simulink model "Simulink_EbolaControlMIMO"  (R2021b)
settings: Solver=VariableStepAuto  StartTime=0.0  StopTime=100  FixedStep=0.0447626744587381  RelTol=1e-3
model workspace (MAT data in the model file):
  Beta = 1.905e-07
  C = 8.015
  Delta = 0.001
  P = 378
  U = 500
  Uu = 250
  V0 = 1.05
  u = 500
undefined symbols (not defined in the file or in its folder): sigbuilder_block
settings Model: Creator=Camilo  LastModifiedBy=Camilo
settings DataIOCC: SaveFormat=Array  OutputTimes=tout

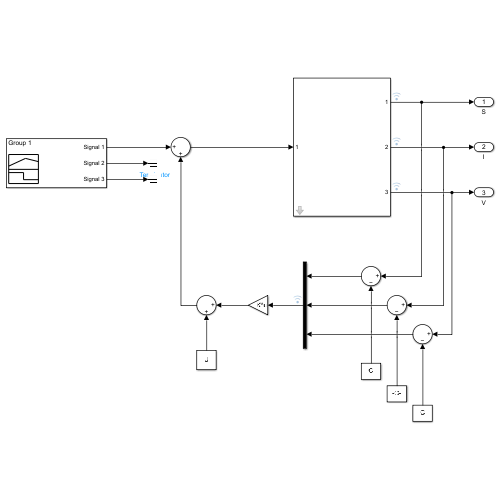
[thumbnail: Simulink's stored preview of the top-level diagram]
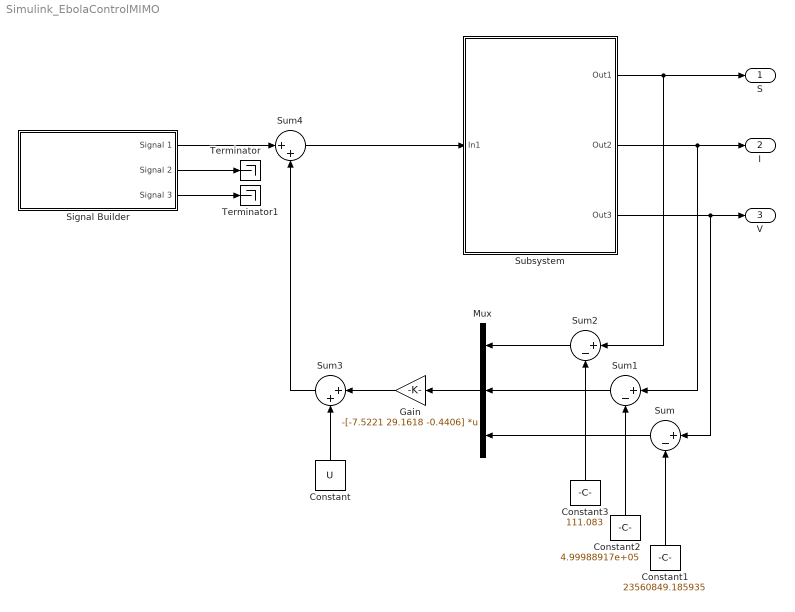
== system Simulink_EbolaControlMIMO ==
  Constant : Constant  Value=U  mask{U=0}
  Constant1 : Constant  Value=23560849.185935
  Constant2 : Constant  Value=4.99988917e+05
  Constant3 : Constant  Value=111.083
  Gain : Gain  Gain=-[-7.5221 29.1618 -0.4406]  Multiplication=Matrix(K*u)
  Mux : Mux  Inputs=3
  Signal Builder : Subsystem  Tag=STV Subsys  LoadFcn=sigbuilder_block('load');  StartFcn=sigbuilder_block('start');  StopFcn=sigbuilder_block('stop');  ClipboardFcn=sigbuilder_block('clipboard');  mask(Sigbuilder block){tuvar=[0:10]}
      mask help: Simulink:masks:SigbuilderBlock_MD
      mask init:
      | if ~strcmp(get_param(bdroot(gcbh),'SimulationStatus'),'stopped') tuvar = sigbuilder_block('maskInit'); end
      settings: CopyFcn=sigbuilder_block('copy');  DeleteFcn=sigbuilder_block('delete');  ModelCloseFcn=sigbuilder_block('modelClose');  PreSaveFcn=sigbuilder_block('preSave');  PauseFcn=sigbuilder_block('pause');  ContinueFcn=sigbuilder_block('continue');  NameChangeFcn=sigbuilder_block('namechange');  OpenFcn=sigbuilder_block('open',[437.6 126.75 619.15 472.45 ]);  CloseFcn=sigbuilder_block('close');
      mask Display: plot(0, 0, 100, 100,[2, 2, 32, 32, 2], [68, 8, 8, 68, 68],[32, 2], [38, 38], [32, 19, 2],[53, 60, 44], [32, 17, 17, 2],[16, 16, 31, 31]);txt = getActiveGroup(gcbh);text(2, 100, txt,'verticalAlignment', 'top');
  Subsystem : Subsystem  mask{V0=23560849.185935, Delta=Delta, P=P, C=C, Beta=Beta}
  Sum : Sum  Inputs=|+-
  Sum1 : Sum  Inputs=|+-
  Sum2 : Sum  Inputs=|+-
  Sum3 : Sum  Inputs=|++
  Sum4 : Sum  Inputs=|++
  Terminator : Terminator
  Terminator1 : Terminator
  S : Outport
  I : Outport  Port=2
  V : Outport  Port=3
  wires:
  Subsystem/2(Out2) -> I/1, Sum1/1
  Subsystem/3(Out3) -> V/1, Sum/1
  Subsystem/1(Out1) -> Sum2/1, S/1
  Constant1/1 -> Sum/2
  Constant2/1 -> Sum1/2
  Constant3/1 -> Sum2/2
  Sum/1 -> Mux/3
  Sum2/1 -> Mux/1
  Sum1/1 -> Mux/2
  Mux/1 -> Gain/1
  Gain/1 -> Sum3/1
  Constant/1 -> Sum3/2
  Sum3/1 -> Sum4/2
  Sum4/1 -> Subsystem/1(In1)
  Signal Builder/1(Signal 1) -> Sum4/1
  Signal Builder/3(Signal 3) -> Terminator1/1
  Signal Builder/2(Signal 2) -> Terminator/1

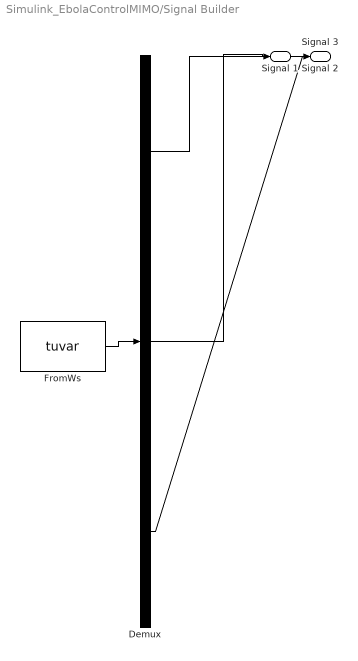
== system Simulink_EbolaControlMIMO/Signal Builder ==
  Demux : Demux  Tag=STV Demux  Outputs=3
      settings: DisplayOption=none
  FromWs : FromWorkspace  Tag=STV FromWs  VariableName=tuvar
      SigBuilderData=|
      | common.afterFinalStr = 'Extrapolate'
      | common.sampleTime = 0
      | dataSet.timeRange = [0 10]
      | dataSet.name = 'Group 1'
      | sbobj.Groups.Name = 'Group 1'
      | sbobj.Groups.Signals(1).Name = 'Signal 1'
      | sbobj.Groups.Signals(1).XData = [0 3 6 6 10]
      | sbobj.Groups.Signals(1).YData = [0.01 0 500 -0.005 0]
      | sbobj.Groups.Signals(2).Name = 'Signal 2'
      | sbobj.Groups.Signals(2).XData = [0 4 4 10]
      | sbobj.Groups.Signals(2).YData = [0 0 500 500]
      | sbobj.Groups.Signals(3).Name = 'Signal 3'
      | sbobj.Groups.Signals(3).XData = [0 4 4 6 6 10]
      | sbobj.Groups.Signals(3).YData = [0 0 500 500 0 0]
  Signal 1 : Outport  Tag=STV Outport
  Signal 2 : Outport  Tag=STV Outport  Port=2
  Signal 3 : Outport  Tag=STV Outport  Port=3
  wires:
  Demux/1 -> Signal 1/1
  FromWs/1 -> Demux/1
  Demux/2 -> Signal 2/1
  Demux/3 -> Signal 3/1

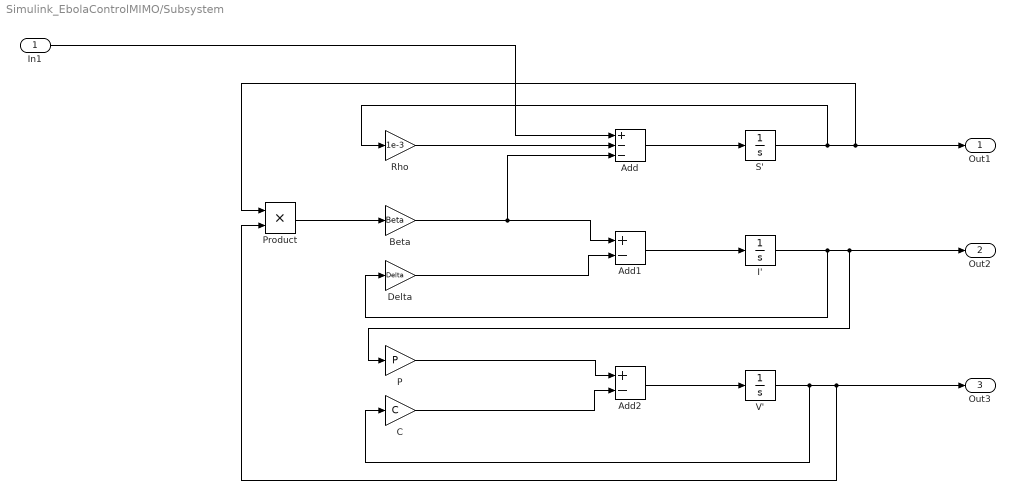
== system Simulink_EbolaControlMIMO/Subsystem ==
  In1 : Inport
  Add : Sum  Inputs=+--
  Add1 : Sum  Inputs=+-
  Add2 : Sum  Inputs=+-
  Beta : Gain  Gain=Beta
  C : Gain  Gain=C
  Delta : Gain  Gain=Delta
  I' : Integrator  InitialCondition=4.99988917e5  LimitOutput=on  LowerSaturationLimit=0
  P : Gain  Gain=P
  Product : Product
  Rho : Gain  Gain=1e-3
  S' : Integrator  InitialCondition=111.083  LimitOutput=on  LowerSaturationLimit=0
  V' : Integrator  InitialCondition=V0  LimitOutput=on  LowerSaturationLimit=0
  Out1 : Outport
  Out2 : Outport  Port=2
  Out3 : Outport  Port=3
  wires:
  Add/1 -> S'/1
  C/1 -> Add2/2
  Beta/1 -> Add1/1, Add/3
  I'/1 -> Out2/1, P/1, Delta/1
  P/1 -> Add2/1
  S'/1 -> Out1/1, Product/1, Rho/1
  Rho/1 -> Add/2
  V'/1 -> Out3/1, Product/2, C/1
  Add2/1 -> V'/1
  Product/1 -> Beta/1
  Add1/1 -> I'/1
  Delta/1 -> Add1/2
  In1/1 -> Add/1
